simulink model "GasExample_V4S"  (R2025b)
settings: Solver=FixedStepAuto  StartTime=0.0  StopTime=1000  FixedStep=0.01  RelTol=1e-3
model workspace (MAT data in the model file):
  alpha = 20
libraries: Bibliothek_FHDO_V1 x23, BibFHDO x20, BibSpielo x11, simulink x9
(part 2 of 2)

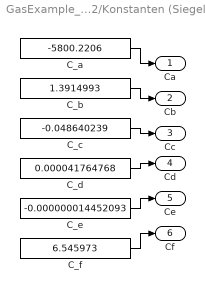
== system GasExample_V4S/Volumen/Befeuchter//Abscheider2/Konstanten (Siegel) ==
  C_a : Constant  Value=-5800.2206
  C_b : Constant  Value=1.3914993
  C_c : Constant  Value=-0.048640239
  C_d : Constant  Value=0.000041764768
  C_e : Constant  Value=-0.000000014452093
  C_f : Constant  Value=6.545973
  Ca : Outport
  Cb : Outport  Port=2
  Cc : Outport  Port=3
  Cd : Outport  Port=4
  Ce : Outport  Port=5
  Cf : Outport  Port=6
  wires:
  C_f/1 -> Cf/1
  C_e/1 -> Ce/1
  C_d/1 -> Cd/1
  C_c/1 -> Cc/1
  C_b/1 -> Cb/1
  C_a/1 -> Ca/1

== system GasExample_V4S/Volumen/Befeuchter//Abscheider2/Normierung auf 1 mol Anteil1 ==
  In1 : Inport
  Mux : Mux
  Product : Product  Inputs=*/  RndMeth=Zero
  Sum of Elements : Sum  Inputs=+
  Switch : Switch  Criteria=u2 > Threshold  SaturateOnIntegerOverflow=off  InputSameDT=off
  Out1 : Outport
  Sum : Outport  Port=2
  wires:
  In1/1 -> Sum of Elements/1, Product/1
  Sum of Elements/1 -> Switch/2, Mux/4, Mux/3, Mux/2, Mux/1, Product/2, Sum/1
  Product/1 -> Switch/1
  Switch/1 -> Out1/1
  Mux/1 -> Switch/3

== system GasExample_V4S/Volumen/Befeuchter//Abscheider2/Normierung auf 1 mol Anteil3 ==
  In1 : Inport
  Mux : Mux
  Product : Product  Inputs=*/  RndMeth=Zero
  Sum of Elements : Sum  Inputs=+
  Switch : Switch  Criteria=u2 > Threshold  SaturateOnIntegerOverflow=off  InputSameDT=off
  Out1 : Outport
  Sum : Outport  Port=2
  wires:
  Mux/1 -> Switch/3
  Switch/1 -> Out1/1
  Product/1 -> Switch/1
  Sum of Elements/1 -> Sum/1, Product/2, Mux/1, Mux/2, Mux/3, Mux/4, Switch/2
  In1/1 -> Product/1, Sum of Elements/1
